simulink model "POWER_factor_correction"  (R2023b)
settings: Solver=VariableStepAuto  StartTime=0.0  StopTime=10  RelTol=1e-3
libraries: spsSeriesRLCBranchLib x4, spsBreakerLib x3, simulink x2, spsACVoltageSourceLib x1, spsCurrentMeasurementLib x1, spsVoltageMeasurementLib x1, sps_lib x1
settings Model: Creator=abdur  LastModifiedBy=abdur

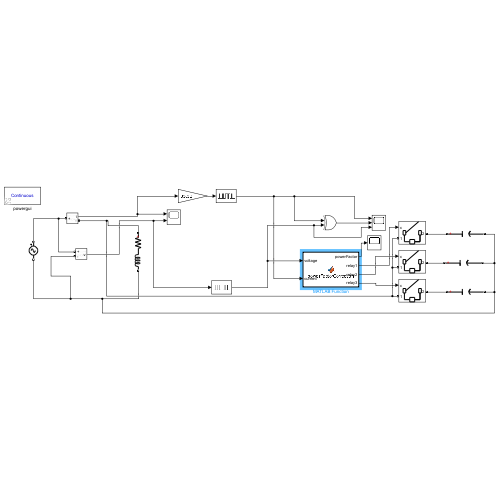
[thumbnail: Simulink's stored preview of the top-level diagram]
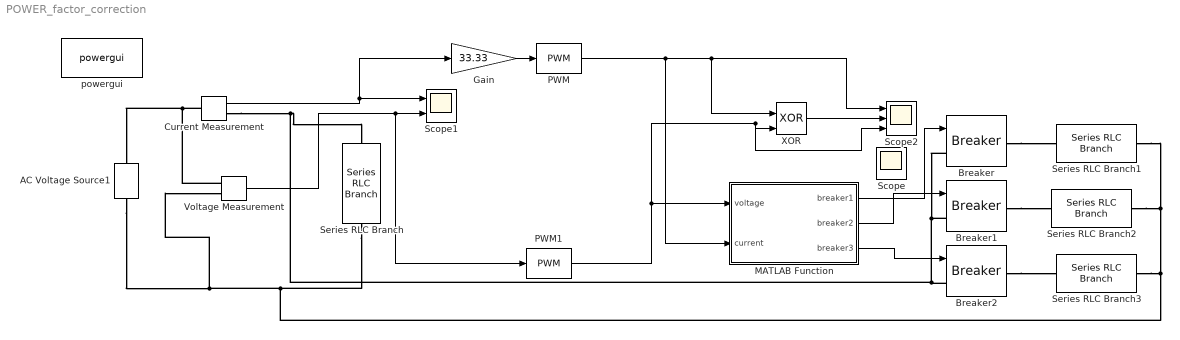
== system POWER_factor_correction ==
  AC Voltage Source1 : spsACVoltageSourceLib/AC Voltage Source  Amplitude=20  Phase=0  Frequency=60  SampleTime=0  Measurements=None  BusType=swing  Pref=10e3  Qref=0  Qmin=-inf  Qmax=+inf
  Breaker : spsBreakerLib/Breaker  InitialState=0  SwitchingTimes="[1/60  5/60]"  External=on  BreakerResistance=0.01  SnubberResistance=1e6  SnubberCapacitance=inf  Measurements=None  MoreParameters=on  NoBreakLoop=off
  Breaker1 : spsBreakerLib/Breaker  InitialState=0  SwitchingTimes="[1/60  5/60]"  External=on  BreakerResistance=0.01  SnubberResistance=1e6  SnubberCapacitance=inf  Measurements=None  MoreParameters=on  NoBreakLoop=off
  Breaker2 : spsBreakerLib/Breaker  InitialState=0  SwitchingTimes="[1/60  5/60]"  External=on  BreakerResistance=0.01  SnubberResistance=1e6  SnubberCapacitance=inf  Measurements=None  MoreParameters=on  NoBreakLoop=off
  Current Measurement : spsCurrentMeasurementLib/Current Measurement  PhasorSimulation=off  OutputType=Complex  PSBequivalent=0
  Gain : Gain  Gain=33.33
  MATLAB Function : MATLAB Function  TreatAsAtomicUnit=on
  PWM : simulink/Discontinuities/PWM  DisableCoverage=on  Period=0.166  InitialDelay=0  DisallowZeroDutyCycle=off  RunAtFixedTimeIntervals=off  SampleTime=0.1
  PWM1 : simulink/Discontinuities/PWM  DisableCoverage=on  Period=0.166  InitialDelay=0  DisallowZeroDutyCycle=off  RunAtFixedTimeIntervals=off  SampleTime=0.1
  Scope : Scope
  Scope1 : Scope  NumInputPorts=2
  Scope2 : Scope  NumInputPorts=3
  Series RLC Branch : spsSeriesRLCBranchLib/Series RLC Branch  LConnTagsString=__new0  RConnTagsString=__new0  BranchType=RL  Resistance=30  Inductance=30e-3  SetiL0=off  InitialCurrent=0  Capacitance=0  Setx0=off  InitialVoltage=0  Measurements=None
  Series RLC Branch1 : spsSeriesRLCBranchLib/Series RLC Branch  LConnTagsString=__new0  RConnTagsString=__new0  BranchType=C  Resistance=0  Inductance=0  SetiL0=off  InitialCurrent=0  Capacitance=47e-6  Setx0=off  InitialVoltage=0  Measurements=None
  Series RLC Branch2 : spsSeriesRLCBranchLib/Series RLC Branch  LConnTagsString=__new0  RConnTagsString=__new0  BranchType=C  Resistance=0  Inductance=0  SetiL0=off  InitialCurrent=0  Capacitance=80e-6  Setx0=off  InitialVoltage=0  Measurements=None
  Series RLC Branch3 : spsSeriesRLCBranchLib/Series RLC Branch  LConnTagsString=__new0  RConnTagsString=__new0  BranchType=C  Resistance=1  Inductance=1e-3  SetiL0=off  InitialCurrent=0  Capacitance=160e-6  Setx0=off  InitialVoltage=0  Measurements=None
  Voltage Measurement : spsVoltageMeasurementLib/Voltage Measurement  PhasorSimulation=off  OutputType=Complex  PSBequivalent=0
  XOR : Logic  Operator=XOR  IconShape=distinctive  AllPortsSameDT=off  OutDataTypeStr=boolean
  powergui : sps_lib/powergui  Priority=1  SimulationMode=Continuous  SampleTime=50e-6  frequency=60  Iterations=50  frequencyindice=60  Pbase=100e6  ErrMax=1e-4  UnitsV=kV  UnitsW=MW  buscounter=0  FunctionMessages=off  echomessages=off  EnableUseOfTLC=off  CurrentSourceSwitches=off  DisableSnubberDevices=off  DisableRonSwitches=off  DisableVfSwitches=off  DisplayEquations=off  AutomaticDiscreteSolvers=off  SolverType=Tustin/Backward Euler (TBE)  Interpol=off  ExternalGateDelay=off  methode=off  Ts=100  x0status=blocks  SPID=on  SwTol=0  HookPort=off  NonlinearTolerance=1e-4  nMaxIteration=100  ContinueOnMaxIteration=off  RestoreLinks=warning  ResistiveCurrentMeasurement=off  Frange=[0:2:500]  Ylog=off  Xlog=on  ShowGrid=off  save=off  variable=ZData  structure=0  ZoomFFT=off  StartTime=0.0  cycles=1  DisplayStyle=1  fundamental=60  FreqAxis=off  MaxFrequency=1000  frequencyindicesteady=1  RmsSteady=1  display=off
  wires:
  Voltage Measurement/1 -> PWM1/1, Scope1/2
  Current Measurement/1 -> Gain/1, Scope1/1
  ? -> Scope/1
  MATLAB Function/1(breaker1) -> Breaker/1
  MATLAB Function/2(breaker2) -> Breaker1/1
  MATLAB Function/3(breaker3) -> Breaker2/1
  Gain/1 -> PWM/1
  PWM/1 -> MATLAB Function/2(current), XOR/1, Scope2/1
  PWM1/1 -> MATLAB Function/1(voltage), Scope2/3, XOR/2
  XOR/1 -> Scope2/2
  connections:
  Current Measurement/RConn1 -- Breaker2/LConn1 -- Breaker/LConn1 -- Breaker1/LConn1 -- Series RLC Branch/LConn1
  Series RLC Branch/RConn1 -- Series RLC Branch2/RConn1 -- Series RLC Branch1/RConn1 -- Series RLC Branch3/RConn1 -- AC Voltage Source1/LConn1 -- Voltage Measurement/LConn2
  Current Measurement/LConn1 -- Voltage Measurement/LConn1 -- AC Voltage Source1/RConn1
  Breaker/RConn1 -- Series RLC Branch1/LConn1
  Breaker1/RConn1 -- Series RLC Branch2/LConn1
  Breaker2/RConn1 -- Series RLC Branch3/LConn1

== matlab function POWER_factor_correction/MATLAB Function ==
  settings: updateMethod=DISCRETE
  data: voltage input; current input; breaker1 output; breaker2 output; breaker3 output
function [ breaker1, breaker2, breaker3] = powerFactorCorrection(voltage, current)
    % Persistent variables to maintain state between function calls
  

    if isempty(timeDifferenceSum)
        timeDifferenceSum = 0;
        sampleCount = 0;
        capState = 0;
        powerFactorSamples = zeros(1, 8);
        capStateSamples = zeros(1, 8);
    end

    % Default values for outputs
    powerFactor = 1;
    breaker1 = 0;
    breaker2 = 0;
    breaker3 = 0;

    % Calculate the time difference between voltage and current zero crossings
    timeDifference = findTimeDifference(voltage, current);

    if ~isempty(timeDifference)
        timeDifferenceSum = timeDifferenceSum + timeDifference;
        sampleCount = sampleCount + 1;
    end

    % Process accumulated time differences
    if sampleCount >= 10
        avgTimeDifference = timeDifferenceSum / sampleCount;
        thetaRad = avgTimeDifference * 2 * pi * 50; % Assuming 50 Hz frequency
        powerFactor = cos(thetaRad);

        % Reset accumulators
        timeDifferenceSum = 0;
        sampleCount = 0;

        % Adjust capacitor state based on power factor
        if powerFactor < 0.95
            capState = min(capState + 1, 7); % Increase capacitance
        elseif powerFactor > 1.05
            capState = max(capState - 1, 0); % Decrease capacitance
        end

        % Store samples for finding optimal power factor
        capStateSamples = circshift(capStateSamples, 1);
        capStateSamples(1) = capState;
        powerFactorSamples = circshift(powerFactorSamples, 1);
        powerFactorSamples(1) = powerFactor;

        % Determine the best capacitor state
        if all(powerFactorSamples)
            [~, bestIndex] = max(powerFactorSamples);
            capState = capStateSamples(bestIndex);
        end

        % Set breaker states based on capacitor state
        [breaker1, breaker2, breaker3] = setBreakers(capState);
    end
end

function timeDifference = findTimeDifference(voltage, current)
    % Placeholder function for finding the time difference between
    % voltage and current zero crossings.
    % Replace with actual implementation.
    timeDifference = rand() * 0.02 - 0.01; % Random value between -0.01 and 0.01
end

function [breaker1, breaker2, breaker3] = setBreakers(capState)
    % Set breaker states based on capacitor state
    switch capState
        case 0
            breaker1 = 0; breaker2 = 0; breaker3 = 0;
        case 1
            breaker1 = 1; breaker2 = 0; breaker3 = 0;
        case 2
            breaker1 = 0; breaker2 = 1; breaker3 = 0;
        case 3
            breaker1 = 1; breaker2 = 1; breaker3 = 0;
        case 4
            breaker1 = 0; breaker2 = 0; breaker3 = 1;
        case 5
            breaker1 = 1; breaker2 = 0; breaker3 = 1;
        case 6
            breaker1 = 0; breaker2 = 1; breaker3 = 1;
        case 7
            breaker1 = 1; breaker2 = 1; breaker3 = 1;
        otherwise
            breaker1 = 0; breaker2 = 0; breaker3 = 0;
    end
end
